simulink model "AOO"  (R2022b)
settings: Solver=FixedStepAuto  StartTime=0.0  StopTime=10.0  FixedStep=1e-3  RelTol=1e-3  EnableMultiTasking=on
undefined symbols (not defined in the file): D10, D11, D12, D2, D5, D8, D9, PTA0, PTA2, PTB9, PTC4, PTD0, PTD2, PTD3
libraries: frdmk64flib x8
settings Model: ExtModeTrigDuration=5  Creator=mutha  LastModifiedBy=mutha
settings SolverCC: AlgebraicLoopSolver=TrustRegion
settings OptimizationCC: EnhancedBackFolding=on  PassReuseOutputArgsAs=Individual arguments  ZeroExternalMemoryAtStartup=off  ZeroInternalMemoryAtStartup=off  MaxStackSize=64  OptimizeBlockOrder=speed  DifferentSizesBufferReuse=on  OptimizationCustomize=off  EfficientTunableParamExpr=on
settings DebuggingCC: ParameterTunabilityLossMsg=error  UnconnectedInputMsg=warning  UnconnectedOutputMsg=warning  UnconnectedLineMsg=warning  SFMachineParentedDataDiag=warning
settings HardwareCC: ProdBitPerPointer=32  ProdBitPerSizeT=32  ProdBitPerPtrDiffT=32  ProdLargestAtomicInteger=Long  ProdLargestAtomicFloat=Double  ProdWordSize=32  ProdHWDeviceType=ARM Compatible->ARM Cortex
settings ModelReferenceCC: EnableRefExpFcnMdlSchedulingChecks=on
settings SFSimCC: MATLABDynamicMemAlloc=off
settings RTWCC: Description=Embedded Coder  SystemTargetFile=ert.tlc  HardwareBoard=NXP FRDM-K64F  TLCOptions="-aInlineSetEventsForThisBaseRateFcn=TLC_FALSE -aSuppressMultiTaskScheduler=TLC_FALSE  -aRateBasedStepFcn=0"  TemplateMakefile=ert_default_tmf  Toolchain=GNU Tools for ARM Embedded Processors  DLArmComputeVersion=19.05
settings CodeAppCC: ForceParamTrailComments=on  IgnoreCustomStorageClasses=off  OperatorAnnotations=on  SimulinkDataObjDesc=on  SFDataObjDesc=on  InsertBlockDesc=on
settings ERTTargetCC: ExtModeTransport=4  ExtModeMexFile=sendToCommService

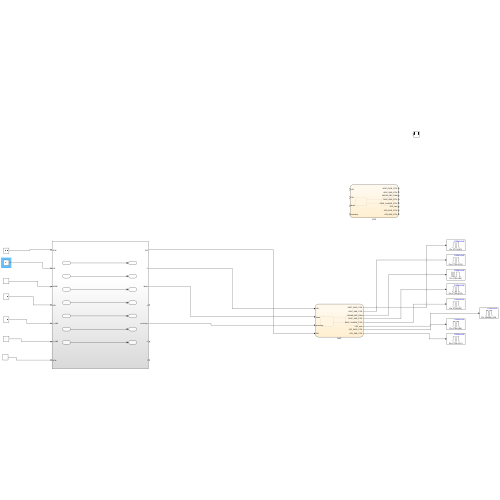
[thumbnail: Simulink's stored preview of the top-level diagram]
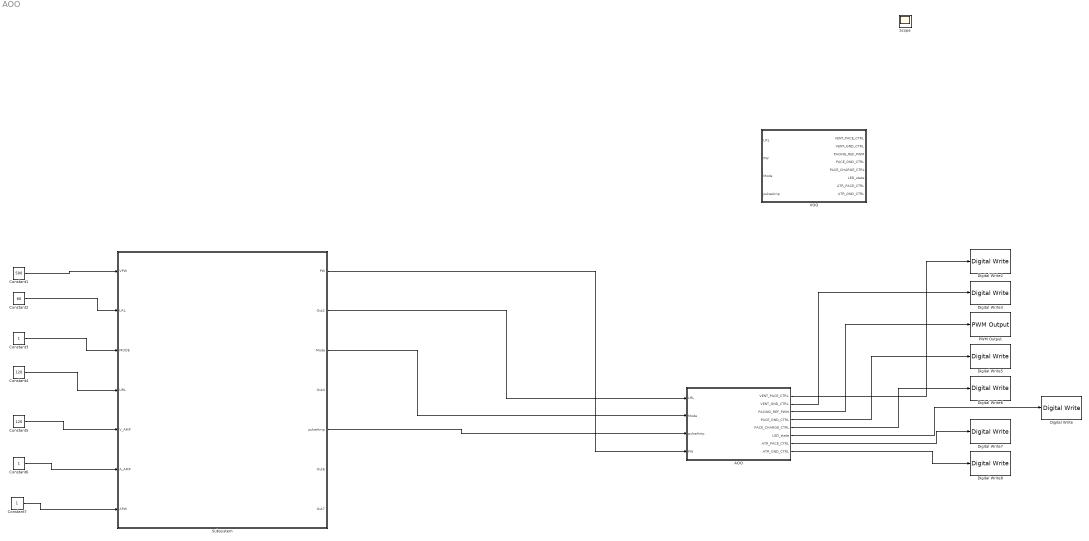
== system AOO ==
  AOO : Stateflow chart  TreatAsAtomicUnit=on
      settings: PortSchema="{\"entries\":[{\"content\":{\"sides\":[{\"content\":{\"connectorIds\":[\"In1\",\"In3\",\"In4\",\"In2\"]},\"type\":\"ConnectorPlacement.EquallySpacedRectSide\",\"uuid\":\"4a9106b9-4977-4ad7-a664-79baeb9488d7\"},{\"content\":{\"connectorIds\":[\"Out1\",\"Out2\",\"Out3\",\"Out4\",\"Out5\",\"Out6\",\"Out7\",\"Out8\"],\"side\":\"RIGHT\"},\"type\":\"ConnectorPlacement.EquallySpacedRectSide\",\"uuid\":\"b9887666-f10a-4603-9f8e-4ad73175cafe\"},{\"content\":{\"connectorIds\":[],\"side\":\"TOP\"},\"type\":\"ConnectorPlacement.EquallySpacedRectSide\",\"uuid\":\"1850edd3-c966-4e07-b98a-67abbc5f02e7\"}]},\"type\":\"ConnectorPlacement.EquallySpacedConnector\",\"uuid\":\"2b9e48c6-c28a-4e83-8c86-f722f9137b29\"}],\"packageUris\":[\"http://schema.mathworks.com/mf0/Connector/R2020b\"],\"version\":\"1.0\"}"
  Constant1 : Constant  Value=500  OutDataTypeStr=int16
  Constant2 : Constant  Value=60  OutDataTypeStr=int16
  Constant3 : Constant  OutDataTypeStr=int8
  Constant4 : Constant  Value=120  OutDataTypeStr=int8
  Constant5 : Constant  Value=120  OutDataTypeStr=int8
  Constant6 : Constant  OutDataTypeStr=int8
  Constant7 : Constant  OutDataTypeStr=int8
  Digital Write : frdmk64flib/Digital Write  Whichpin=GREEN_LED
  Digital Write2 : frdmk64flib/Digital Write  Whichpin=PTC4 (D9)
  Digital Write3 : frdmk64flib/Digital Write  Whichpin=PTD3 (D12)
  Digital Write5 : frdmk64flib/Digital Write  Whichpin=PTD0 (D10)
  Digital Write6 : frdmk64flib/Digital Write  Whichpin=PTB9 (D2)
  Digital Write7 : frdmk64flib/Digital Write  Whichpin=PTA0 (D8)
  Digital Write8 : frdmk64flib/Digital Write  Whichpin=PTD2 (D11)
  PWM Output : frdmk64flib/PWM Output  Whichpin=PTA2 (D5)  InitialFrequency=2000  InitialDutyCycle=100
  Scope : Scope
  Subsystem : Subsystem
  VOO : Stateflow chart  TreatAsAtomicUnit=on
  wires:
  Constant1/1 -> Subsystem/1(VPW)
  Constant2/1 -> Subsystem/2(LRL)
  Constant3/1 -> Subsystem/3(MODE)
  Constant4/1 -> Subsystem/4(URL)
  Constant5/1 -> Subsystem/5(V_AMP)
  Constant7/1 -> Subsystem/7(APW)
  Constant6/1 -> Subsystem/6(A_AMP)
  Subsystem/3(Mode) -> AOO/3(Mode)
  Subsystem/2(Out2) -> AOO/1(LRL)
  AOO/8(ATR_GND_CTRL) -> Digital Write8/1
  AOO/7(ATR_PACE_CTRL) -> Digital Write7/1
  AOO/6(LED_state) -> Digital Write/1
  AOO/5(PACE_CHARGE_CTRL) -> Digital Write6/1
  AOO/4(PACE_GND_CTRL) -> Digital Write5/1
  AOO/3(PACING_REF_PWM) -> PWM Output/1
  AOO/2(VENT_GND_CTRL) -> Digital Write3/1
  AOO/1(VENT_PACE_CTRL) -> Digital Write2/1
  Subsystem/1(PW) -> AOO/2(PW)
  Subsystem/5(pulseAmp) -> AOO/4(pulseAmp)

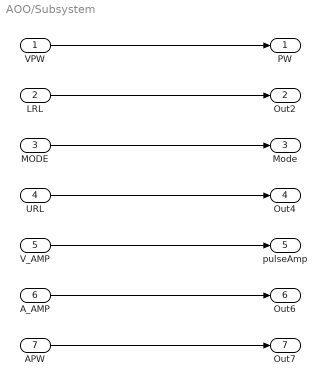
== system AOO/Subsystem ==
  VPW : Inport
  LRL : Inport  Port=2  OutDataTypeStr=int16
  MODE : Inport  Port=3
  URL : Inport  Port=4
  V_AMP : Inport  Port=5
  A_AMP : Inport  Port=6
  APW : Inport  Port=7
  PW : Outport
  Out2 : Outport  Port=2
  Mode : Outport  Port=3
  Out4 : Outport  Port=4
  pulseAmp : Outport  Port=5
  Out6 : Outport  Port=6
  Out7 : Outport  Port=7
  wires:
  VPW/1 -> PW/1
  LRL/1 -> Out2/1
  MODE/1 -> Mode/1
  URL/1 -> Out4/1
  V_AMP/1 -> pulseAmp/1
  A_AMP/1 -> Out6/1
  APW/1 -> Out7/1

== stateflow chart AOO/AOO ==
  state LED_on%State2(VOO)
    %Discharging C22
    PACE_CHARGE_CTRL = false;
    PACE_GND_CTRL = true;
    VENT_PACE_CTRL = false;
    ATR_PACE_CTRL = true;
    VENT_GND_CTRL = true; %not sure
    ATR_GND_CTRL = false;
    %LED STATE
    LED_state = true;
  state LED_off %State 1(VOO)
    %Charging C22
    %Mode = 2;
    PACING_REF_PWM = (pulseAmp / 5);
    PACE_CHARGE_CTRL = true;
    VENT_PACE_CTRL = false;
    ATR_PACE_CTRL = false;
    %Discharging C21
    PACE_GND_CTRL = true;
    VENT_GND_CTRL = false;
    ATR_GND_CTRL = true;
    %LED STATE
    LED_state = false;
  (default) -> LED_off %State 1(VOO)
  LED_off %State 1(VOO) -> LED_on%State2(VOO) : after (PW,msec)
  LED_on%State2(VOO) -> LED_off %State 1(VOO) : after ((60000/LRL) - PW, msec)
  data: VENT_PACE_CTRL output boolean; VENT_GND_CTRL output boolean; PACING_REF_PWM output int8; PACE_GND_CTRL output boolean; PACE_CHARGE_CTRL output boolean; LED_state output boolean; ATR_PACE_CTRL output boolean; ATR_GND_CTRL output boolean; LRL input int16; PW input int16; Mode input int8; pulseAmp input int8

== stateflow chart AOO/VOO ==
  state LED_off %State 1(VOO)
    entry:
    %Mode = 1;
    %Charging C22
    PACING_REF_PWM = (pulseAmp / 5);
    PACE_CHARGE_CTRL = true;
    VENT_PACE_CTRL = false;
    ATR_PACE_CTRL = false;
    %Discharging C21
    PACE_GND_CTRL = true;
    VENT_GND_CTRL = true;
    ATR_GND_CTRL = false;
    %LED STATE
    LED_state = false;
  state LED_on%State2(VOO)
    entry:
    %Mode = 1;
    %Discharging C22
    PACE_CHARGE_CTRL = false;
    PACE_GND_CTRL = true;
    VENT_PACE_CTRL = true;
    ATR_PACE_CTRL = false;
    VENT_GND_CTRL = false;
    ATR_GND_CTRL = true; %not sure
    %LED STATE
    LED_state = true;
  (default) -> LED_off %State 1(VOO)
  LED_off %State 1(VOO) -> LED_on%State2(VOO) : after (PW,msec)
  LED_on%State2(VOO) -> LED_off %State 1(VOO) : after (((60000/LRL)-PW), msec)
  data: VENT_PACE_CTRL output boolean; VENT_GND_CTRL output boolean; PACING_REF_PWM output int8; PACE_GND_CTRL output boolean; PACE_CHARGE_CTRL output boolean; LED_state output boolean; ATR_PACE_CTRL output boolean; ATR_GND_CTRL output boolean; LRL input int16; PW input int16; Mode input; pulseAmp input int8
